simulink model "AAI"  (R2022b)
settings: Solver=FixedStepAuto  StartTime=0.0  StopTime=10.0  FixedStep=1e-3  RelTol=1e-3  EnableMultiTasking=on
undefined symbols (not defined in the file): D0, D10, D11, D12, D13, D2, D5, D6, D8, D9, PTA0, PTA2, PTB9, PTC16, PTC2, PTC4, PTD0, PTD1, PTD2, PTD3
libraries: frdmk64flib x10
settings Model: ExtModeTrigDuration=5  Creator=Ali Umar  LastModifiedBy=seankhaira
settings OptimizationCC: EnhancedBackFolding=on  PassReuseOutputArgsAs=Individual arguments  ZeroExternalMemoryAtStartup=off  ZeroInternalMemoryAtStartup=off  MaxStackSize=64  OptimizeBlockOrder=speed  DifferentSizesBufferReuse=on  OptimizationCustomize=off  EfficientTunableParamExpr=on
settings DebuggingCC: ParameterTunabilityLossMsg=error
settings HardwareCC: ProdBitPerPointer=32  ProdBitPerSizeT=32  ProdBitPerPtrDiffT=32  ProdLargestAtomicInteger=Long  ProdLargestAtomicFloat=Double  ProdWordSize=32  ProdHWDeviceType=ARM Compatible->ARM Cortex
settings SFSimCC: MATLABDynamicMemAlloc=off
settings RTWCC: Description=Embedded Coder  SystemTargetFile=ert.tlc  HardwareBoard=NXP FRDM-K64F  TLCOptions="-aInlineSetEventsForThisBaseRateFcn=TLC_FALSE -aSuppressMultiTaskScheduler=TLC_FALSE  -aRateBasedStepFcn=0"  TemplateMakefile=ert_default_tmf  Toolchain=GNU Tools for ARM Embedded Processors
settings CodeAppCC: ForceParamTrailComments=on  IgnoreCustomStorageClasses=off  OperatorAnnotations=on  SimulinkDataObjDesc=on  SFDataObjDesc=on  InsertBlockDesc=on
settings ERTTargetCC: ExtModeTransport=4  ExtModeMexFile=sendToCommService

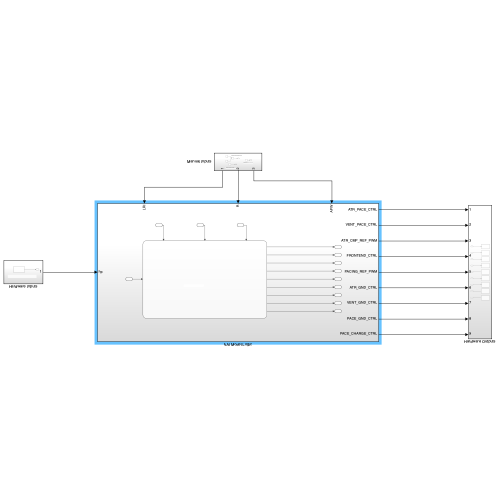
[thumbnail: Simulink's stored preview of the top-level diagram]
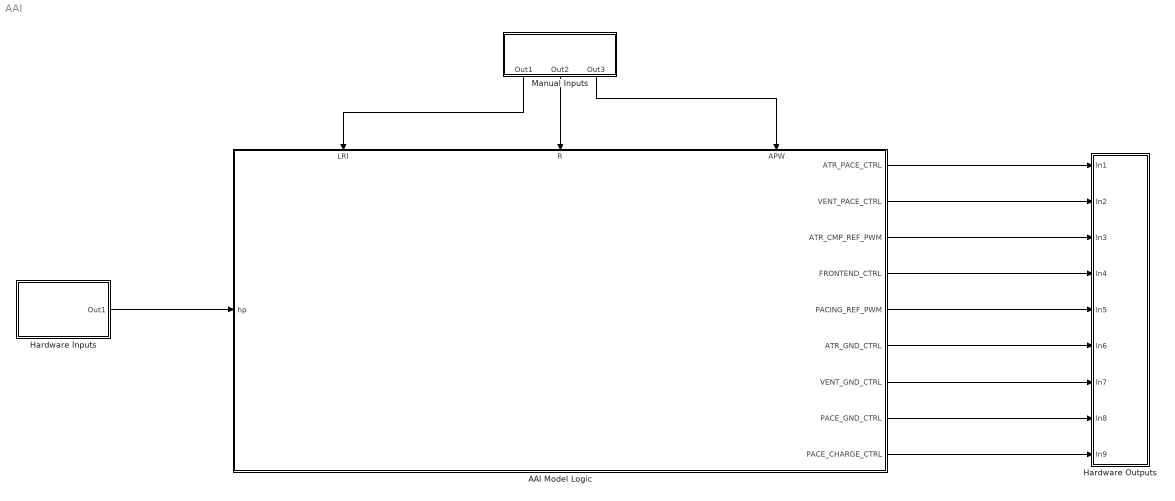
== system AAI ==
  AAI Model Logic : Subsystem
      settings: PortSchema="{\"entries\":[{\"content\":{\"sides\":[{\"content\":{\"connectorIds\":[\"In1\"]},\"type\":\"ConnectorPlacement.EquallySpacedRectSide\",\"uuid\":\"69aa4b1d-c490-42a5-9d07-618761886ad3\"},{\"content\":{\"connectorIds\":[\"Out1\",\"Out2\",\"Out3\",\"Out4\",\"Out5\",\"Out6\",\"Out7\",\"Out8\",\"Out9\"],\"side\":\"RIGHT\"},\"type\":\"ConnectorPlacement.EquallySpacedRectSide\",\"uuid\":\"7290674e-c6cc-413b-813c-95b8013b7049\"},{\"content\":{\"connectorIds\":[\"In2\",\"In3\",\"In4\"],\"side\":\"TOP\"},\"type\":\"ConnectorPlacement.EquallySpacedRectSide\",\"uuid\":\"3d44994f-4a3f-4e78-8559-6d18ad10a943\"}]},\"type\":\"ConnectorPlacement.EquallySpacedConnector\",\"uuid\":\"ec0bfab0-e8bf-4e06-813d-ed65cf4e8f94\"}],\"packageUris\":[\"http://schema.mathworks.com/mf0/Connector/R2020b\"],\"version\":\"1.0\"}"
  Hardware Inputs : Subsystem
  Hardware Outputs : Subsystem
  Manual Inputs : Subsystem
  wires:
  Manual Inputs/2(Out2) -> AAI Model Logic/3(R)
  Manual Inputs/3(Out3) -> AAI Model Logic/4(APW)
  Hardware Inputs/1(Out1) -> AAI Model Logic/1(hp)
  AAI Model Logic/1(ATR_PACE_CTRL) -> Hardware Outputs/1(In1)
  AAI Model Logic/2(VENT_PACE_CTRL) -> Hardware Outputs/2(In2)
  AAI Model Logic/3(ATR_CMP_REF_PWM) -> Hardware Outputs/3(In3)
  AAI Model Logic/4(FRONTEND_CTRL) -> Hardware Outputs/4(In4)
  AAI Model Logic/5(PACING_REF_PWM) -> Hardware Outputs/5(In5)
  AAI Model Logic/6(ATR_GND_CTRL) -> Hardware Outputs/6(In6)
  AAI Model Logic/8(PACE_GND_CTRL) -> Hardware Outputs/8(In8)
  AAI Model Logic/7(VENT_GND_CTRL) -> Hardware Outputs/7(In7)
  AAI Model Logic/9(PACE_CHARGE_CTRL) -> Hardware Outputs/9(In9)
  Manual Inputs/1(Out1) -> AAI Model Logic/2(LRI)

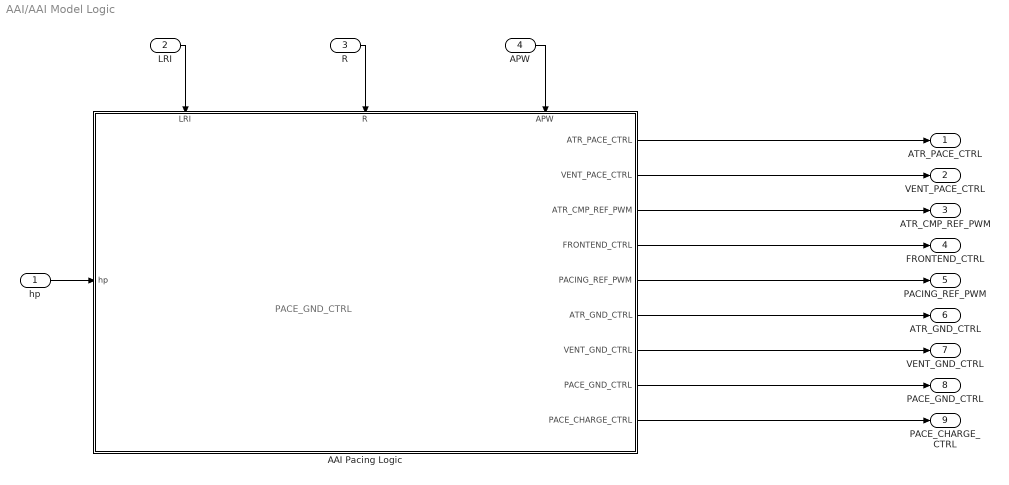
== system AAI/AAI Model Logic ==
  note: PACE_GND_CTRL
  hp : Inport
  LRI : Inport  Port=2
  R : Inport  Port=3
  APW : Inport  Port=4
  AAI Pacing Logic : Stateflow chart  TreatAsAtomicUnit=on
      settings: PortSchema="{\"entries\":[{\"content\":{\"sides\":[{\"content\":{\"connectorIds\":[\"In4\"]},\"type\":\"ConnectorPlacement.EquallySpacedRectSide\",\"uuid\":\"2fbd3f15-98aa-43f7-a7cc-cc8317656681\"},{\"content\":{\"connectorIds\":[\"Out1\",\"Out2\",\"Out3\",\"Out4\",\"Out5\",\"Out6\",\"Out8\",\"Out7\",\"Out9\"],\"side\":\"RIGHT\"},\"type\":\"ConnectorPlacement.EquallySpacedRectSide\",\"uuid\":\"6ca9ce92-abfb-4dfe-8dc1-b8c2756ce902\"},{\"content\":{\"connectorIds\":[\"In1\",\"In2\",\"In3\"],\"side\":\"TOP\"},\"type\":\"ConnectorPlacement.EquallySpacedRectSide\",\"uuid\":\"afdd4081-cdfe-440c-b70f-a33f5b30e5b5\"},{\"content\":{\"connectorIds\":[],\"side\":\"BOTTOM\"},\"type\":\"ConnectorPlacement.EquallySpacedRectSide\",\"uuid\":\"5f031f29-572e-497e-89db-cdc1cd9f1a52\"}]},\"type\":\"ConnectorPlacement.EquallySpacedConnector\",\"uuid\":\"38f9d585-7dff-40ee-9c0b-6e56b8b4fe59\"}],\"packageUris\":[\"http://schema.mathworks.com/mf0/Connector/R2020b\"],\"version\":\"1.0\"}"
  ATR_PACE_CTRL : Outport
  VENT_PACE_CTRL : Outport  Port=2
  ATR_CMP_REF_PWM : Outport  Port=3
  FRONTEND_CTRL : Outport  Port=4
  PACING_REF_PWM : Outport  Port=5
  ATR_GND_CTRL : Outport  Port=6
  VENT_GND_CTRL : Outport  Port=7
  PACE_GND_CTRL : Outport  Port=8
  PACE_CHARGE_CTRL : Outport  Port=9
  wires:
  AAI Pacing Logic/2(VENT_PACE_CTRL) -> VENT_PACE_CTRL/1
  hp/1 -> AAI Pacing Logic/4(hp)
  LRI/1 -> AAI Pacing Logic/1(LRI)
  AAI Pacing Logic/3(ATR_CMP_REF_PWM) -> ATR_CMP_REF_PWM/1
  R/1 -> AAI Pacing Logic/2(R)
  AAI Pacing Logic/5(PACING_REF_PWM) -> PACING_REF_PWM/1
  AAI Pacing Logic/8(VENT_GND_CTRL) -> VENT_GND_CTRL/1
  AAI Pacing Logic/1(ATR_PACE_CTRL) -> ATR_PACE_CTRL/1
  APW/1 -> AAI Pacing Logic/3(APW)
  AAI Pacing Logic/9(PACE_CHARGE_CTRL) -> PACE_CHARGE_CTRL/1
  AAI Pacing Logic/7(PACE_GND_CTRL) -> PACE_GND_CTRL/1
  AAI Pacing Logic/6(ATR_GND_CTRL) -> ATR_GND_CTRL/1
  AAI Pacing Logic/4(FRONTEND_CTRL) -> FRONTEND_CTRL/1

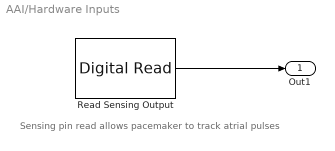
== system AAI/Hardware Inputs ==
  note: Sensing pin read allows pacemaker to track atrial pulses
  Read Sensing Output : frdmk64flib/Digital Read  Whichpin=PTC16 (D0)  SampleTime=-1
  Out1 : Outport
  wires:
  Read Sensing Output/1 -> Out1/1

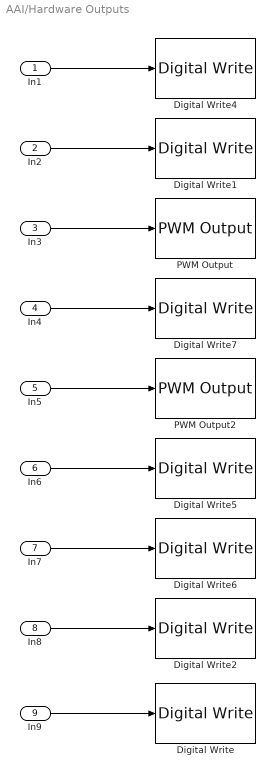
== system AAI/Hardware Outputs ==
  In1 : Inport
  In2 : Inport  Port=2
  In3 : Inport  Port=3
  In4 : Inport  Port=4
  In5 : Inport  Port=5
  In6 : Inport  Port=6
  In7 : Inport  Port=7
  In8 : Inport  Port=8
  In9 : Inport  Port=9
  Digital Write : frdmk64flib/Digital Write  Whichpin=PTB9 (D2)
  Digital Write1 : frdmk64flib/Digital Write  Whichpin=PTC4 (D9)
  Digital Write2 : frdmk64flib/Digital Write  Whichpin=PTD0 (D10)
  Digital Write4 : frdmk64flib/Digital Write  Whichpin=PTA0 (D8)
  Digital Write5 : frdmk64flib/Digital Write  Whichpin=PTD2 (D11)
  Digital Write6 : frdmk64flib/Digital Write  Whichpin=PTD3 (D12)
  Digital Write7 : frdmk64flib/Digital Write  Whichpin=PTD1 (D13)
  PWM Output : frdmk64flib/PWM Output  Whichpin=PTC2 (D6)  InitialFrequency=2000  InitialDutyCycle=50
  PWM Output2 : frdmk64flib/PWM Output  Whichpin=PTA2 (D5)  InitialFrequency=2000  InitialDutyCycle=50
  wires:
  In7/1 -> Digital Write6/1
  In2/1 -> Digital Write1/1
  In6/1 -> Digital Write5/1
  In1/1 -> Digital Write4/1
  In4/1 -> Digital Write7/1
  In5/1 -> PWM Output2/1
  In9/1 -> Digital Write/1
  In3/1 -> PWM Output/1
  In8/1 -> Digital Write2/1

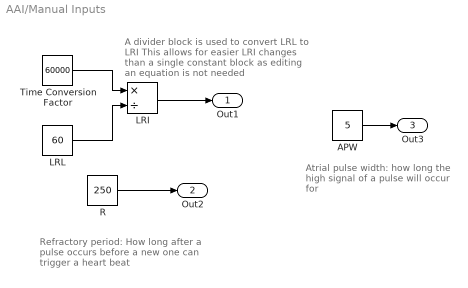
== system AAI/Manual Inputs ==
  note: Atrial pulse width: how long the high signal of
      | a pulse will occur for
  note: Refractory period: How long after a pulse occurs before a new one can trigger a heart beat
  note: A divider block is used to convert LRL to LRI
      | This allows for easier LRI changes than a single constant block as editing an equation is not needed
  APW : Constant  Value=5
  LRI : Product  Inputs=*/
  LRL : Constant  Value=60
  R : Constant  Value=250
  Time Conversion Factor : Constant  Value=60000
  Out1 : Outport
  Out2 : Outport  Port=2
  Out3 : Outport  Port=3
  wires:
  R/1 -> Out2/1
  APW/1 -> Out3/1
  LRL/1 -> LRI/2
  LRI/1 -> Out1/1
  Time Conversion Factor/1 -> LRI/1

== stateflow chart AAI/AAI Model Logic/AAI Pacing Logic ==
  state Pacing
    entry:
    PACE_CHARGE_CTRL = false;
    PACE_GND_CTRL = true;
    VENT_PACE_CTRL = false;
    ATR_GND_CTRL = false;
    VENT_GND_CTRL = false;
    ATR_PACE_CTRL = true;
  note: Pacing state discharges the pacing capacitor for an APW amount of time
  note: If on startup, if there is no pulse felt for LRI time, a pace will occur
  state Flatline_Startup_Check
    entry:
    %Turn sensing on to start
    FRONTEND_CTRL = true;
    ATR_CMP_REF_PWM = 75;
    %Charging C22
    ATR_PACE_CTRL = false;
    VENT_PACE_CTRL = false;
    PACING_REF_PWM  = 75;
    PACE_CHARGE_CTRL = true;
    %Discharging Backwards Capacitor
    PACE_GND_CTRL = true;
    VENT_PACE_CTRL = false;
    ATR_PACE_CTRL = false;
    VENT_GND_CTRL = false;
    ATR_GND_CTRL = true;
  note: On power on, turn on sensing, charge pacing capacitor, discharge backwards capacitor
  note: No refractory wait on startup, as the initial time is not connected to a pulse, and so there is no need to wait a refractory period to allow pulses to be considered.
      |
      | No refractory wait for the first pulse solves the likely start case of a pulse being sensed immediately, but being ignored as it fell within
      | a wrong refractory period
  note: To avoid false positives with the sensing circuit, it is turned off during refractory waiting
      | (this was disabled due to causing bugs in heartview)
  state Refractory_Safety
    entry:
    %Turn sensing off to avoid errors
    %FRONTEND_CTRL = false;
    %VENT_CMP_REF_PWM = 75;
    %Charging C22
    ATR_PACE_CTRL = false;
    VENT_PACE_CTRL = false;
    PACING_REF_PWM  = 75;
    PACE_CHARGE_CTRL = true;
    %Discharging Backwards Capacitor
    PACE_GND_CTRL = true;
    VENT_PACE_CTRL = false;
    ATR_PACE_CTRL = false;
    VENT_GND_CTRL = false;
    ATR_GND_CTRL = true;
  note: This state occurs after a pulse, so the pacing capacitor is charged
      | and the backwards capacitor is discharged
      |
      | No issues with continually charging the capacitors even if the heart naturally pulsed instead of the pacemaker, as the capacitors will only hold the required charge
  note: The above state always occurs after a pulse (natural or pace) has occured
      | Thus, here it is allowed to always wait a refractory period
  note: If the heart pulsed before the LRI - R time, then no need to pace, go back to waiting the refractory period
  note: The prior state always occurs after the refractory
      | period of a pulse, and thus the longest time allowed
      | before a LRI pulse should be sent is LRI - R
      |
      | If no pulse felt for that duration, pacing is activated
  state After_Refractory_Check
    entry:
    %Turn sensing on to start loop
    FRONTEND_CTRL = true;
    ATR_CMP_REF_PWM = 75;
  Flatline_Startup_Check -> Pacing [order 1] : after(LRI,msec)
  After_Refractory_Check -> Pacing [order 1] : after(LRI-R,msec)
  (default) -> Flatline_Startup_Check
  Pacing -> Refractory_Safety : after(APW,msec)
  Flatline_Startup_Check -> Refractory_Safety [order 2] : [hp==true]
  After_Refractory_Check -> Refractory_Safety [order 2] : [hp==true]
  Refractory_Safety -> After_Refractory_Check : after(R,msec)
  data: ATR_PACE_CTRL output; VENT_PACE_CTRL output; ATR_CMP_REF_PWM output; FRONTEND_CTRL output; PACING_REF_PWM output; ATR_GND_CTRL output; PACE_GND_CTRL output; VENT_GND_CTRL output; LRI input; R input; APW input; hp input; PACE_CHARGE_CTRL output
